simulink model "gm_hybrid_lht_vnl"  (R2019b)
settings: Solver=FixedStepDiscrete  StartTime=0.0  StopTime=inf  FixedStep=1/120e6  RelTol=1e-3
undefined symbols (not defined in the file or in its folder): bt, height, nTheta, width
libraries: hdlsllib x632, simulink x518, hdlmdlgenlib x7, dspsrcs4 x1
(part 2 of 18)

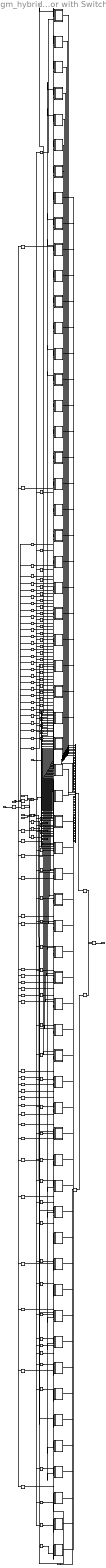
== system gm_hybrid_lht_vnl/Hybrid LHT/Hybrid LHT Accumulator/Accumulator with Switches ==
  shift : Inport  OutDataTypeStr=fixdt(0, 6, 0)  PortDimensions=[1 60]  SampleTime=8.33333333333333e-09
  hough_address : Inport  Port=2  OutDataTypeStr=fixdt(0, 11, 0)  PortDimensions=[1 60]  SampleTime=8.33333333333333e-09
  edge : Inport  Port=3  OutDataTypeStr=boolean  PortDimensions=1  SampleTime=8.33333333333333e-09
  mode : Inport  Port=4  OutDataTypeStr=boolean  PortDimensions=1  SampleTime=8.33333333333333e-09
  read_address : Inport  Port=5  OutDataTypeStr=uint16  PortDimensions=1  SampleTime=8.33333333333333e-09
  clear : Inport  Port=6  OutDataTypeStr=boolean  PortDimensions=1  SampleTime=8.33333333333333e-09
  theta_index : Inport  Port=7  OutDataTypeStr=uint16  PortDimensions=1  SampleTime=8.33333333333333e-09
  Accumulator_instance1 : Subsystem
  Accumulator_instance10 : Subsystem
  Accumulator_instance11 : Subsystem
  Accumulator_instance12 : Subsystem
  Accumulator_instance13 : Subsystem
  Accumulator_instance14 : Subsystem
  Accumulator_instance15 : Subsystem
  Accumulator_instance16 : Subsystem
  Accumulator_instance17 : Subsystem
  Accumulator_instance18 : Subsystem
  Accumulator_instance19 : Subsystem
  Accumulator_instance2 : Subsystem
  Accumulator_instance20 : Subsystem
  Accumulator_instance21 : Subsystem
  Accumulator_instance22 : Subsystem
  Accumulator_instance23 : Subsystem
  Accumulator_instance24 : Subsystem
  Accumulator_instance25 : Subsystem
  Accumulator_instance26 : Subsystem
  Accumulator_instance27 : Subsystem
  Accumulator_instance28 : Subsystem
  Accumulator_instance29 : Subsystem
  Accumulator_instance3 : Subsystem
  Accumulator_instance30 : Subsystem
  Accumulator_instance31 : Subsystem
  Accumulator_instance32 : Subsystem
  Accumulator_instance33 : Subsystem
  Accumulator_instance34 : Subsystem
  Accumulator_instance35 : Subsystem
  Accumulator_instance36 : Subsystem
  Accumulator_instance37 : Subsystem
  Accumulator_instance38 : Subsystem
  Accumulator_instance39 : Subsystem
  Accumulator_instance4 : Subsystem
  Accumulator_instance40 : Subsystem
  Accumulator_instance41 : Subsystem
  Accumulator_instance42 : Subsystem
  Accumulator_instance43 : Subsystem
  Accumulator_instance44 : Subsystem
  Accumulator_instance45 : Subsystem
  Accumulator_instance46 : Subsystem
  Accumulator_instance47 : Subsystem
  Accumulator_instance48 : Subsystem
  Accumulator_instance49 : Subsystem
  Accumulator_instance5 : Subsystem
  Accumulator_instance50 : Subsystem
  Accumulator_instance51 : Subsystem
  Accumulator_instance52 : Subsystem
  Accumulator_instance53 : Subsystem
  Accumulator_instance54 : Subsystem
  Accumulator_instance55 : Subsystem
  Accumulator_instance56 : Subsystem
  Accumulator_instance57 : Subsystem
  Accumulator_instance58 : Subsystem
  Accumulator_instance59 : Subsystem
  Accumulator_instance6 : Subsystem
  Accumulator_instance60 : Subsystem
  Accumulator_instance7 : Subsystem
  Accumulator_instance8 : Subsystem
  Accumulator_instance9 : Subsystem
  Data Type Conversion : DataTypeConversion  OutDataTypeStr=fixdt(0, 11, 0)  SampleTime=8.33333333333333e-09
  Delay : Delay  DelayLength=double(1)  InitialCondition=0  SampleTime=8.33333333333333e-09
  Multiport Switch1 : MultiPortSwitch  DataPortOrder=Zero-based contiguous  Inputs=2  DiagnosticForDefault=None  zeroidx=on  SampleTime=8.33333333333333e-09
  Selector : Selector  NumberOfDimensions=2  IndexMode=Zero-based  SampleTime=8.33333333333333e-09  IndexOptions=Index vector (dialog),Index vector (port)  Indices=double(0),double(0)  OutputSizes=double(1),double(1)
  Switch : Switch  Criteria=u2 > Threshold  Threshold=double(0)  OutDataTypeStr=fixdt(0, 11, 0)  SampleTime=8.33333333333333e-09
  delayMatch{,1..122} (123 alike) : Delay  DelayLength=double(2)  InitialCondition=0  SampleTime=8.33333333333333e-09
  t : Demux  Outputs=60
  t1 : Demux  Outputs=60
  t2 : Concatenate  NumInputs=60
  t3 : Reshape  OutputDimensionality=Row vector (2-D)
  hps : Outport
  wires:
  Delay/1 -> delayMatch122/1
  Multiport Switch1/1 -> delayMatch3/1, delayMatch5/1, delayMatch7/1, delayMatch9/1, delayMatch11/1, delayMatch13/1, delayMatch15/1, delayMatch17/1, delayMatch19/1, delayMatch21/1, delayMatch23/1, delayMatch25/1, delayMatch27/1, delayMatch29/1, delayMatch31/1, delayMatch33/1, delayMatch35/1, delayMatch37/1, delayMatch39/1, delayMatch41/1, delayMatch43/1, delayMatch45/1, delayMatch47/1, delayMatch49/1, delayMatch51/1, delayMatch53/1, delayMatch55/1, delayMatch57/1, delayMatch59/1, delayMatch61/1, delayMatch63/1, delayMatch65/1, delayMatch67/1, delayMatch69/1, delayMatch71/1, delayMatch73/1, delayMatch75/1, delayMatch77/1, delayMatch79/1, delayMatch81/1, delayMatch83/1, delayMatch85/1, delayMatch87/1, delayMatch89/1, delayMatch91/1, delayMatch93/1, delayMatch95/1, delayMatch97/1, delayMatch99/1, delayMatch101/1, delayMatch103/1, delayMatch105/1, delayMatch107/1, delayMatch109/1, delayMatch111/1, delayMatch113/1, delayMatch115/1, delayMatch117/1, delayMatch119/1, delayMatch121/1
  delayMatch121/1 -> Accumulator_instance60/4(edge)
  delayMatch120/1 -> Accumulator_instance60/2(mode)
  delayMatch119/1 -> Accumulator_instance59/4(edge)
  delayMatch118/1 -> Accumulator_instance59/2(mode)
  delayMatch117/1 -> Accumulator_instance58/4(edge)
  delayMatch116/1 -> Accumulator_instance58/2(mode)
  delayMatch115/1 -> Accumulator_instance57/4(edge)
  delayMatch114/1 -> Accumulator_instance57/2(mode)
  delayMatch113/1 -> Accumulator_instance56/4(edge)
  delayMatch112/1 -> Accumulator_instance56/2(mode)
  delayMatch111/1 -> Accumulator_instance55/4(edge)
  delayMatch110/1 -> Accumulator_instance55/2(mode)
  delayMatch109/1 -> Accumulator_instance54/4(edge)
  delayMatch108/1 -> Accumulator_instance54/2(mode)
  delayMatch107/1 -> Accumulator_instance53/4(edge)
  delayMatch106/1 -> Accumulator_instance53/2(mode)
  delayMatch105/1 -> Accumulator_instance52/4(edge)
  delayMatch104/1 -> Accumulator_instance52/2(mode)
  delayMatch103/1 -> Accumulator_instance51/4(edge)
  delayMatch102/1 -> Accumulator_instance51/2(mode)
  delayMatch101/1 -> Accumulator_instance50/4(edge)
  delayMatch100/1 -> Accumulator_instance50/2(mode)
  delayMatch99/1 -> Accumulator_instance49/4(edge)
  delayMatch98/1 -> Accumulator_instance49/2(mode)
  delayMatch97/1 -> Accumulator_instance48/4(edge)
  delayMatch96/1 -> Accumulator_instance48/2(mode)
  delayMatch95/1 -> Accumulator_instance47/4(edge)
  delayMatch94/1 -> Accumulator_instance47/2(mode)
  delayMatch93/1 -> Accumulator_instance46/4(edge)
  delayMatch92/1 -> Accumulator_instance46/2(mode)
  delayMatch91/1 -> Accumulator_instance45/4(edge)
  delayMatch90/1 -> Accumulator_instance45/2(mode)
  delayMatch89/1 -> Accumulator_instance44/4(edge)
  delayMatch88/1 -> Accumulator_instance44/2(mode)
  delayMatch87/1 -> Accumulator_instance43/4(edge)
  delayMatch86/1 -> Accumulator_instance43/2(mode)
  delayMatch85/1 -> Accumulator_instance42/4(edge)
  delayMatch84/1 -> Accumulator_instance42/2(mode)
  delayMatch83/1 -> Accumulator_instance41/4(edge)
  delayMatch82/1 -> Accumulator_instance41/2(mode)
  delayMatch81/1 -> Accumulator_instance40/4(edge)
  delayMatch80/1 -> Accumulator_instance40/2(mode)
  delayMatch79/1 -> Accumulator_instance39/4(edge)
  delayMatch78/1 -> Accumulator_instance39/2(mode)
  delayMatch77/1 -> Accumulator_instance38/4(edge)
  delayMatch76/1 -> Accumulator_instance38/2(mode)
  delayMatch75/1 -> Accumulator_instance37/4(edge)
  delayMatch74/1 -> Accumulator_instance37/2(mode)
  delayMatch73/1 -> Accumulator_instance36/4(edge)
  delayMatch72/1 -> Accumulator_instance36/2(mode)
  delayMatch71/1 -> Accumulator_instance35/4(edge)
  delayMatch70/1 -> Accumulator_instance35/2(mode)
  delayMatch69/1 -> Accumulator_instance34/4(edge)
  delayMatch68/1 -> Accumulator_instance34/2(mode)
  delayMatch67/1 -> Accumulator_instance33/4(edge)
  delayMatch66/1 -> Accumulator_instance33/2(mode)
  delayMatch65/1 -> Accumulator_instance32/4(edge)
  delayMatch64/1 -> Accumulator_instance32/2(mode)
  delayMatch63/1 -> Accumulator_instance31/4(edge)
  delayMatch62/1 -> Accumulator_instance31/2(mode)
  delayMatch61/1 -> Accumulator_instance30/4(edge)
  delayMatch60/1 -> Accumulator_instance30/2(mode)
  delayMatch59/1 -> Accumulator_instance29/4(edge)
  delayMatch58/1 -> Accumulator_instance29/2(mode)
  delayMatch57/1 -> Accumulator_instance28/4(edge)
  delayMatch56/1 -> Accumulator_instance28/2(mode)
  delayMatch55/1 -> Accumulator_instance27/4(edge)
  delayMatch54/1 -> Accumulator_instance27/2(mode)
  delayMatch53/1 -> Accumulator_instance26/4(edge)
  delayMatch52/1 -> Accumulator_instance26/2(mode)
  delayMatch51/1 -> Accumulator_instance25/4(edge)
  delayMatch50/1 -> Accumulator_instance25/2(mode)
  delayMatch49/1 -> Accumulator_instance24/4(edge)
  delayMatch48/1 -> Accumulator_instance24/2(mode)
  delayMatch47/1 -> Accumulator_instance23/4(edge)
  delayMatch46/1 -> Accumulator_instance23/2(mode)
  delayMatch45/1 -> Accumulator_instance22/4(edge)
  delayMatch44/1 -> Accumulator_instance22/2(mode)
  delayMatch43/1 -> Accumulator_instance21/4(edge)
  delayMatch42/1 -> Accumulator_instance21/2(mode)
  delayMatch41/1 -> Accumulator_instance20/4(edge)
  delayMatch40/1 -> Accumulator_instance20/2(mode)
  delayMatch39/1 -> Accumulator_instance19/4(edge)
  delayMatch38/1 -> Accumulator_instance19/2(mode)
  delayMatch37/1 -> Accumulator_instance18/4(edge)
  delayMatch36/1 -> Accumulator_instance18/2(mode)
  delayMatch35/1 -> Accumulator_instance17/4(edge)
  delayMatch34/1 -> Accumulator_instance17/2(mode)
  delayMatch33/1 -> Accumulator_instance16/4(edge)
  delayMatch32/1 -> Accumulator_instance16/2(mode)
  delayMatch31/1 -> Accumulator_instance15/4(edge)
  delayMatch30/1 -> Accumulator_instance15/2(mode)
  delayMatch29/1 -> Accumulator_instance14/4(edge)
  delayMatch28/1 -> Accumulator_instance14/2(mode)
  delayMatch27/1 -> Accumulator_instance13/4(edge)
  delayMatch26/1 -> Accumulator_instance13/2(mode)
  delayMatch25/1 -> Accumulator_instance12/4(edge)
  delayMatch24/1 -> Accumulator_instance12/2(mode)
  delayMatch23/1 -> Accumulator_instance11/4(edge)
  delayMatch22/1 -> Accumulator_instance11/2(mode)
  delayMatch21/1 -> Accumulator_instance10/4(edge)
  delayMatch20/1 -> Accumulator_instance10/2(mode)
  delayMatch19/1 -> Accumulator_instance9/4(edge)
  delayMatch18/1 -> Accumulator_instance9/2(mode)
  delayMatch17/1 -> Accumulator_instance8/4(edge)
  delayMatch16/1 -> Accumulator_instance8/2(mode)
  delayMatch15/1 -> Accumulator_instance7/4(edge)
  delayMatch14/1 -> Accumulator_instance7/2(mode)
  delayMatch13/1 -> Accumulator_instance6/4(edge)
  delayMatch12/1 -> Accumulator_instance6/2(mode)
  delayMatch11/1 -> Accumulator_instance5/4(edge)
  delayMatch10/1 -> Accumulator_instance5/2(mode)
  delayMatch9/1 -> Accumulator_instance4/4(edge)
  delayMatch8/1 -> Accumulator_instance4/2(mode)
  delayMatch7/1 -> Accumulator_instance3/4(edge)
  delayMatch6/1 -> Accumulator_instance3/2(mode)
  delayMatch5/1 -> Accumulator_instance2/4(edge)
  delayMatch4/1 -> Accumulator_instance2/2(mode)
  Data Type Conversion/1 -> delayMatch1/1
  delayMatch2/1 -> Accumulator_instance1/2(mode)
  theta_index/1 -> Delay/1
  clear/1 -> Multiport Switch1/2
  read_address/1 -> Data Type Conversion/1
  mode/1 -> Multiport Switch1/1, delayMatch/1, delayMatch2/1, delayMatch4/1, delayMatch6/1, delayMatch8/1, delayMatch10/1, delayMatch12/1, delayMatch14/1, delayMatch16/1, delayMatch18/1, delayMatch20/1, delayMatch22/1, delayMatch24/1, delayMatch26/1, delayMatch28/1, delayMatch30/1, delayMatch32/1, delayMatch34/1, delayMatch36/1, delayMatch38/1, delayMatch40/1, delayMatch42/1, delayMatch44/1, delayMatch46/1, delayMatch48/1, delayMatch50/1, delayMatch52/1, delayMatch54/1, delayMatch56/1, delayMatch58/1, delayMatch60/1, delayMatch62/1, delayMatch64/1, delayMatch66/1, delayMatch68/1, delayMatch70/1, delayMatch72/1, delayMatch74/1, delayMatch76/1, delayMatch78/1, delayMatch80/1, delayMatch82/1, delayMatch84/1, delayMatch86/1, delayMatch88/1, delayMatch90/1, delayMatch92/1, delayMatch94/1, delayMatch96/1, delayMatch98/1, delayMatch100/1, delayMatch102/1, delayMatch104/1, delayMatch106/1, delayMatch108/1, delayMatch110/1, delayMatch112/1, delayMatch114/1, delayMatch116/1, delayMatch118/1, delayMatch120/1
  edge/1 -> Multiport Switch1/3
  hough_address/1 -> Switch/1
  shift/1 -> t/1
  Accumulator_instance60/1(hps) -> t2/60
  Accumulator_instance59/1(hps) -> t2/59
  Accumulator_instance58/1(hps) -> t2/58
  Accumulator_instance57/1(hps) -> t2/57
  Accumulator_instance56/1(hps) -> t2/56
  Accumulator_instance55/1(hps) -> t2/55
  Accumulator_instance54/1(hps) -> t2/54
  Accumulator_instance53/1(hps) -> t2/53
  Accumulator_instance52/1(hps) -> t2/52
  Accumulator_instance51/1(hps) -> t2/51
  Accumulator_instance50/1(hps) -> t2/50
  Accumulator_instance49/1(hps) -> t2/49
  Accumulator_instance48/1(hps) -> t2/48
  Accumulator_instance47/1(hps) -> t2/47
  Accumulator_instance46/1(hps) -> t2/46
  Accumulator_instance45/1(hps) -> t2/45
  Accumulator_instance44/1(hps) -> t2/44
  Accumulator_instance43/1(hps) -> t2/43
  Accumulator_instance42/1(hps) -> t2/42
  Accumulator_instance41/1(hps) -> t2/41
  Accumulator_instance40/1(hps) -> t2/40
  Accumulator_instance39/1(hps) -> t2/39
  Accumulator_instance38/1(hps) -> t2/38
  Accumulator_instance37/1(hps) -> t2/37
  Accumulator_instance36/1(hps) -> t2/36
  Accumulator_instance35/1(hps) -> t2/35
  Accumulator_instance34/1(hps) -> t2/34
  Accumulator_instance33/1(hps) -> t2/33
  Accumulator_instance32/1(hps) -> t2/32
  Accumulator_instance31/1(hps) -> t2/31
  Accumulator_instance30/1(hps) -> t2/30
  Accumulator_instance29/1(hps) -> t2/29
  Accumulator_instance28/1(hps) -> t2/28
  Accumulator_instance27/1(hps) -> t2/27
  Accumulator_instance26/1(hps) -> t2/26
  Accumulator_instance25/1(hps) -> t2/25
  Accumulator_instance24/1(hps) -> t2/24
  Accumulator_instance23/1(hps) -> t2/23
  Accumulator_instance22/1(hps) -> t2/22
  Accumulator_instance21/1(hps) -> t2/21
  Accumulator_instance20/1(hps) -> t2/20
  Accumulator_instance19/1(hps) -> t2/19
  Accumulator_instance18/1(hps) -> t2/18
  Accumulator_instance17/1(hps) -> t2/17
  Accumulator_instance16/1(hps) -> t2/16
  Accumulator_instance15/1(hps) -> t2/15
  Accumulator_instance14/1(hps) -> t2/14
  Accumulator_instance13/1(hps) -> t2/13
  Accumulator_instance12/1(hps) -> t2/12
  Accumulator_instance11/1(hps) -> t2/11
  Accumulator_instance10/1(hps) -> t2/10
  Accumulator_instance9/1(hps) -> t2/9
  Accumulator_instance8/1(hps) -> t2/8
  Accumulator_instance7/1(hps) -> t2/7
  Accumulator_instance6/1(hps) -> t2/6
  Accumulator_instance5/1(hps) -> t2/5
  Accumulator_instance4/1(hps) -> t2/4
  Accumulator_instance3/1(hps) -> t2/3
  Accumulator_instance2/1(hps) -> t2/2
  Accumulator_instance1/1(hps) -> t2/1
  t2/1 -> t3/1
  t1/60 -> Accumulator_instance60/3(address)
  t1/59 -> Accumulator_instance59/3(address)
  t1/58 -> Accumulator_instance58/3(address)
  t1/57 -> Accumulator_instance57/3(address)
  t1/56 -> Accumulator_instance56/3(address)
  t1/55 -> Accumulator_instance55/3(address)
  t1/54 -> Accumulator_instance54/3(address)
  t1/53 -> Accumulator_instance53/3(address)
  t1/52 -> Accumulator_instance52/3(address)
  t1/51 -> Accumulator_instance51/3(address)
  t1/50 -> Accumulator_instance50/3(address)
  t1/49 -> Accumulator_instance49/3(address)
  t1/48 -> Accumulator_instance48/3(address)
  t1/47 -> Accumulator_instance47/3(address)
  t1/46 -> Accumulator_instance46/3(address)
  t1/45 -> Accumulator_instance45/3(address)
  t1/44 -> Accumulator_instance44/3(address)
  t1/43 -> Accumulator_instance43/3(address)
  t1/42 -> Accumulator_instance42/3(address)
  t1/41 -> Accumulator_instance41/3(address)
  t1/40 -> Accumulator_instance40/3(address)
  t1/39 -> Accumulator_instance39/3(address)
  t1/38 -> Accumulator_instance38/3(address)
  t1/37 -> Accumulator_instance37/3(address)
  t1/36 -> Accumulator_instance36/3(address)
  t1/35 -> Accumulator_instance35/3(address)
  t1/34 -> Accumulator_instance34/3(address)
  t1/33 -> Accumulator_instance33/3(address)
  t1/32 -> Accumulator_instance32/3(address)
  t1/31 -> Accumulator_instance31/3(address)
  t1/30 -> Accumulator_instance30/3(address)
  t1/29 -> Accumulator_instance29/3(address)
  t1/28 -> Accumulator_instance28/3(address)
  t1/27 -> Accumulator_instance27/3(address)
  t1/26 -> Accumulator_instance26/3(address)
  t1/25 -> Accumulator_instance25/3(address)
  t1/24 -> Accumulator_instance24/3(address)
  t1/23 -> Accumulator_instance23/3(address)
  t1/22 -> Accumulator_instance22/3(address)
  t1/21 -> Accumulator_instance21/3(address)
  t1/20 -> Accumulator_instance20/3(address)
  t1/19 -> Accumulator_instance19/3(address)
  t1/18 -> Accumulator_instance18/3(address)
  t1/17 -> Accumulator_instance17/3(address)
  t1/16 -> Accumulator_instance16/3(address)
  t1/15 -> Accumulator_instance15/3(address)
  t1/14 -> Accumulator_instance14/3(address)
  t1/13 -> Accumulator_instance13/3(address)
  t1/12 -> Accumulator_instance12/3(address)
  t1/11 -> Accumulator_instance11/3(address)
  t1/10 -> Accumulator_instance10/3(address)
  t1/9 -> Accumulator_instance9/3(address)
  t1/8 -> Accumulator_instance8/3(address)
  t1/7 -> Accumulator_instance7/3(address)
  t1/6 -> Accumulator_instance6/3(address)
  t1/5 -> Accumulator_instance5/3(address)
  t1/4 -> Accumulator_instance4/3(address)
  t1/3 -> Accumulator_instance3/3(address)
  t1/2 -> Accumulator_instance2/3(address)
  t1/1 -> Accumulator_instance1/3(address)
  t/60 -> Accumulator_instance60/1(shift)
  t/59 -> Accumulator_instance59/1(shift)
  t/58 -> Accumulator_instance58/1(shift)
  t/57 -> Accumulator_instance57/1(shift)
  t/56 -> Accumulator_instance56/1(shift)
  t/55 -> Accumulator_instance55/1(shift)
  t/54 -> Accumulator_instance54/1(shift)
  t/53 -> Accumulator_instance53/1(shift)
  t/52 -> Accumulator_instance52/1(shift)
  t/51 -> Accumulator_instance51/1(shift)
  t/50 -> Accumulator_instance50/1(shift)
  t/49 -> Accumulator_instance49/1(shift)
  t/48 -> Accumulator_instance48/1(shift)
  t/47 -> Accumulator_instance47/1(shift)
  t/46 -> Accumulator_instance46/1(shift)
  t/45 -> Accumulator_instance45/1(shift)
  t/44 -> Accumulator_instance44/1(shift)
  t/43 -> Accumulator_instance43/1(shift)
  t/42 -> Accumulator_instance42/1(shift)
  t/41 -> Accumulator_instance41/1(shift)
  t/40 -> Accumulator_instance40/1(shift)
  t/39 -> Accumulator_instance39/1(shift)
  t/38 -> Accumulator_instance38/1(shift)
  t/37 -> Accumulator_instance37/1(shift)
  t/36 -> Accumulator_instance36/1(shift)
  t/35 -> Accumulator_instance35/1(shift)
  t/34 -> Accumulator_instance34/1(shift)
  t/33 -> Accumulator_instance33/1(shift)
  t/32 -> Accumulator_instance32/1(shift)
  t/31 -> Accumulator_instance31/1(shift)
  t/30 -> Accumulator_instance30/1(shift)
  t/29 -> Accumulator_instance29/1(shift)
  t/28 -> Accumulator_instance28/1(shift)
  t/27 -> Accumulator_instance27/1(shift)
  t/26 -> Accumulator_instance26/1(shift)
  t/25 -> Accumulator_instance25/1(shift)
  t/24 -> Accumulator_instance24/1(shift)
  t/23 -> Accumulator_instance23/1(shift)
  t/22 -> Accumulator_instance22/1(shift)
  t/21 -> Accumulator_instance21/1(shift)
  t/20 -> Accumulator_instance20/1(shift)
  t/19 -> Accumulator_instance19/1(shift)
  t/18 -> Accumulator_instance18/1(shift)
  t/17 -> Accumulator_instance17/1(shift)
  t/16 -> Accumulator_instance16/1(shift)
  t/15 -> Accumulator_instance15/1(shift)
  t/14 -> Accumulator_instance14/1(shift)
  t/13 -> Accumulator_instance13/1(shift)
  t/12 -> Accumulator_instance12/1(shift)
  t/11 -> Accumulator_instance11/1(shift)
  t/10 -> Accumulator_instance10/1(shift)
  t/9 -> Accumulator_instance9/1(shift)
  t/8 -> Accumulator_instance8/1(shift)
  t/7 -> Accumulator_instance7/1(shift)
  t/6 -> Accumulator_instance6/1(shift)
  t/5 -> Accumulator_instance5/1(shift)
  t/4 -> Accumulator_instance4/1(shift)
  t/3 -> Accumulator_instance3/1(shift)
  t/2 -> Accumulator_instance2/1(shift)
  t/1 -> Accumulator_instance1/1(shift)
  Switch/1 -> t1/1
  Selector/1 -> hps/1
  delayMatch3/1 -> Accumulator_instance1/4(edge)
  delayMatch122/1 -> Selector/2
  delayMatch1/1 -> Switch/3
  t3/1 -> Selector/1
  delayMatch/1 -> Switch/2

== system gm_hybrid_lht_vnl/Hybrid LHT/Hybrid LHT Kernel/Extract Active Votes ==
  note: Check the indices to ensure they are in the correct limits
  Theta : Inport  OutDataTypeStr=uint8  PortDimensions=1  SampleTime=8.33333333333333e-09
  Add : Sum  AccumDataTypeStr=fixdt(1, 10, 0)  OutDataTypeStr=fixdt(1, 10, 0)  SampleTime=8.33333333333333e-09
  Add1 : Sum  Inputs=+-  AccumDataTypeStr=fixdt(1, 12, 0)  OutDataTypeStr=fixdt(1, 12, 0)  SampleTime=8.33333333333333e-09
  Add2 : Sum  Inputs=+-  AccumDataTypeStr=fixdt(1, 9, 0)  OutDataTypeStr=fixdt(1, 9, 0)  SampleTime=8.33333333333333e-09
  Add3 : Sum  AccumDataTypeStr=fixdt(1, 11, 0)  OutDataTypeStr=fixdt(1, 11, 0)  SampleTime=8.33333333333333e-09
  Add4 : Sum  Inputs=+-  AccumDataTypeStr=uint8  OutDataTypeStr=uint8  SampleTime=8.33333333333333e-09
  Constant : Constant  Value=[-30 -29 -28 -27 -26 -25 -24 -23 -22 -21 -20 -19 -18 -17 -16 -15 -14 -13 -12 -11 -10 -9 -8 -7 -6 -5 -4 -3 -2 -1 0 1 2 3 4 5 6 7 8 9 10 11 12 13 14 15 16 17 18 19 20 21 22 23 24 25 26 27 28 29]  VectorParams1D=off  OutDataTypeStr=fixdt(1, 6, 0)  SampleTime=-1
  Data Type Conversion : DataTypeConversion  OutDataTypeStr=uint8  SampleTime=8.33333333333333e-09
  Data Type Conversion1 : DataTypeConversion  OutDataTypeStr=uint8  SampleTime=8.33333333333333e-09
  Gain1 : Product  Inputs=**  OutDataTypeStr=uint8  SampleTime=8.33333333333333e-09
  Gain1_const : Constant  Value=60  OutDataTypeStr=uint8  SampleTime=-1
  GetShift : Subsystem
  High : Constant  Value=59  OutDataTypeStr=uint8  SampleTime=-1
  High1 : Constant  Value=59  OutDataTypeStr=uint8  SampleTime=-1
  Low : Constant  Value=0  OutDataTypeStr=fixdt(0, 1, 0)  SampleTime=-1
  Multiport Switch2 : MultiPortSwitch  DataPortOrder=Zero-based contiguous  Inputs=2  DiagnosticForDefault=None  zeroidx=on  OutDataTypeStr=fixdt(1, 11, 0)  SampleTime=8.33333333333333e-09
  Multiport Switch3 : MultiPortSwitch  DataPortOrder=Zero-based contiguous  Inputs=2  DiagnosticForDefault=None  zeroidx=on  OutDataTypeStr=fixdt(1, 12, 0)  SampleTime=8.33333333333333e-09
  PipelineRegister : Delay  DelayLength=double(1)  InitialCondition=0  SampleTime=8.33333333333333e-09
  Relational : RelationalOperator  Operator=<  OutDataTypeStr=boolean  SampleTime=8.33333333333333e-09  RndMeth=Nearest
  Relational1 : RelationalOperator  Operator=>  OutDataTypeStr=boolean  SampleTime=8.33333333333333e-09  RndMeth=Nearest
  Selector4 : Selector  NumberOfDimensions=2  IndexMode=Zero-based  SampleTime=8.33333333333333e-09  IndexOptions=Index vector (dialog),Index vector (dialog)  Indices=double(0),double([59 58 57 56 55 54 53 52 51 50 49 48 47 46 45 44 43 42 41 40 39 38 37 36 35 34 33 32 31 30 29 28 27 26 25 24 23 22 21 20 19 18 17 16 15 14 13 12 11 10 9 8 7 6 5 4 3 2 1 0])  OutputSizes=double(1),double(1)
  delayMatch : Delay  DelayLength=double(1)  InitialCondition=0  SampleTime=8.33333333333333e-09
  nTheta : Constant  Value=60  OutDataTypeStr=uint8  SampleTime=-1
  Index : Outport  VectorParamsAs1DForOutWhenUnconnected=off
  wires:
  Gain1/1 -> PipelineRegister/1
  Theta/1 -> GetShift/1(Theta), delayMatch/1
  Gain1_const/1 -> Gain1/1
  nTheta/1 -> Add1/2, Add3/2
  Selector4/1 -> Index/1
  Relational1/1 -> Multiport Switch3/1
  Relational/1 -> Multiport Switch2/1
  Multiport Switch3/1 -> Data Type Conversion/1
  Multiport Switch2/1 -> Add1/1, Multiport Switch3/2, Relational1/1
  Low/1 -> Relational/2
  High1/1 -> Add4/1
  High/1 -> Relational1/2
  GetShift/1(Shift) -> Gain1/2
  PipelineRegister/1 -> Add2/2
  Data Type Conversion1/1 -> Add4/2
  Data Type Conversion/1 -> Data Type Conversion1/1
  Constant/1 -> Add/2
  Add4/1 -> Selector4/1
  Add3/1 -> Multiport Switch2/3
  Add2/1 -> Add/1
  Add1/1 -> Multiport Switch3/3
  Add/1 -> Add3/1, Multiport Switch2/2, Relational/1
  delayMatch/1 -> Add2/1

== system gm_hybrid_lht_vnl/Hybrid LHT/Hybrid LHT Kernel/Gradient Kernel System ==
  Edge : Inport  OutDataTypeStr=fixdt(0, 1, 0)  PortDimensions=1  SampleTime=8.33333333333333e-09
  X : Inport  Port=2  OutDataTypeStr=fixdt(1, 11, 0)  PortDimensions=1  SampleTime=8.33333333333333e-09
  Y : Inport  Port=3  OutDataTypeStr=fixdt(1, 10, 0)  PortDimensions=1  SampleTime=8.33333333333333e-09
  Theta : Inport  Port=4  OutDataTypeStr=uint8  PortDimensions=1  SampleTime=8.33333333333333e-09
  Get Index and Fix Limits : Subsystem
  Hough Kernel : Subsystem
  vEdge : Outport  VectorParamsAs1DForOutWhenUnconnected=off
  Rho : Outport  Port=2  VectorParamsAs1DForOutWhenUnconnected=off
  Shift : Outport  Port=3  VectorParamsAs1DForOutWhenUnconnected=off
  wires:
  Theta/1 -> Get Index and Fix Limits/1(Theta)
  Y/1 -> Hough Kernel/3(Y)
  X/1 -> Hough Kernel/2(X)
  Edge/1 -> Hough Kernel/1(Edge)
  Hough Kernel/2(Rho) -> Rho/1
  Hough Kernel/1(vEdge) -> vEdge/1
  Get Index and Fix Limits/2(Shift) -> Shift/1
  Get Index and Fix Limits/1(Index) -> Hough Kernel/4(Index)

== system gm_hybrid_lht_vnl/Hybrid LHT_vnl/Hybrid LHT Accumulator/Accumulator with Switches ==
  shift : Inport
  hough_address : Inport  Port=2
  edge : Inport  Port=3
  mode : Inport  Port=4
  read_address : Inport  Port=5
  clear : Inport  Port=6
  theta_index : Inport  Port=7
  Accumulator : Subsystem
  Data Type Conversion : DataTypeConversion  OutDataTypeStr=fixdt(0,ceil(log2(maxRho*2)),0)
  Delay : Delay  DelayLength=1
  Multiport Switch1 : MultiPortSwitch  DataPortOrder=Zero-based contiguous  Inputs=2  zeroidx=on
  Selector : Selector  NumberOfDimensions=2  IndexMode=Zero-based  InputPortWidth=3  IndexOptions=Index vector (dialog),Index vector (port)  Indices=0,0  OutputSizes=1,1
  Switch : Switch  Criteria=u2 > Threshold
  hps : Outport
  wires:
  shift/1 -> Accumulator/1(shift)
  Accumulator/1(hps) -> Selector/1
  mode/1 -> Switch/2, Multiport Switch1/1, Accumulator/2(mode)
  read_address/1 -> Data Type Conversion/1
  Switch/1 -> Accumulator/3(address)
  Multiport Switch1/1 -> Accumulator/4(edge)
  hough_address/1 -> Switch/1
  theta_index/1 -> Delay/1
  Selector/1 -> hps/1
  edge/1 -> Multiport Switch1/3
  clear/1 -> Multiport Switch1/2
  Data Type Conversion/1 -> Switch/3
  Delay/1 -> Selector/2

== system gm_hybrid_lht_vnl/Hybrid LHT_vnl/Hybrid LHT Kernel/Extract Active Votes ==
  note: Check the indices to ensure they are in the correct limits
  Theta : Inport
  Add : Sum
  Add1 : Sum  Inputs=+-
  Add2 : Sum  Inputs=+-
  Add3 : Sum
  Add4 : Sum  Inputs=+-  OutDataTypeStr=uint8
  Constant : Constant  Value=[-lambda:1:lambda-subflag]  VectorParams1D=off  OutDataTypeStr=fixdt(1,ceil(log2(lambda+1))+1, 0)  SampleTime=-1
  Data Type Conversion : DataTypeConversion  OutDataTypeStr=fixdt(0, ceil(log2(nTheta+1)), 0)
  Data Type Conversion1 : DataTypeConversion  OutDataTypeStr=uint8
  Gain1 : Gain  Gain=nTheta/L  ParamDataTypeStr=fixdt(0, ceil(log2(nTheta+1)), 0)  OutDataTypeStr=fixdt(0, ceil(log2(nTheta+1)), 0)
  GetShift : Subsystem
  High : Constant  Value=nTheta/L-1  OutDataTypeStr=fixdt(0,ceil(log2(nTheta)),0)  SampleTime=-1
  High1 : Constant  Value=nTheta/L-1  OutDataTypeStr=fixdt(0,ceil(log2(nTheta)),0)  SampleTime=-1
  Low : Constant  Value=0  OutDataTypeStr=fixdt(0,1,0)  SampleTime=-1
  Multiport Switch2 : MultiPortSwitch  DataPortOrder=Zero-based contiguous  Inputs=2  zeroidx=on
  Multiport Switch3 : MultiPortSwitch  DataPortOrder=Zero-based contiguous  Inputs=2  zeroidx=on
  Relational : RelationalOperator  Operator=<  OutDataTypeStr=boolean  RndMeth=Nearest
  Relational1 : RelationalOperator  Operator=>  OutDataTypeStr=boolean  RndMeth=Nearest
  Selector4 : Selector  NumberOfDimensions=2  IndexMode=Zero-based  InputPortWidth=3  IndexOptions=Index vector (dialog),Index vector (dialog)  Indices=0,[nTheta/floor(36/ceil(log2(2*maxRho)))-1:-1:0]  OutputSizes=1,1
  nTheta : Constant  Value=nTheta/L  OutDataTypeStr=fixdt(0,ceil(log2(nTheta+1)),0)  SampleTime=-1
  Index : Outport  VectorParamsAs1DForOutWhenUnconnected=off
  wires:
  Gain1/1 -> Add2/2
  GetShift/1(Shift) -> Gain1/1
  Selector4/1 -> Index/1
  Constant/1 -> Add/2
  Add1/1 -> Multiport Switch3/3
  Relational/1 -> Multiport Switch2/1
  Multiport Switch3/1 -> Data Type Conversion/1
  High/1 -> Relational1/2
  Relational1/1 -> Multiport Switch3/1
  Add3/1 -> Multiport Switch2/3
  Low/1 -> Relational/2
  Multiport Switch2/1 -> Add1/1, Relational1/1, Multiport Switch3/2
  nTheta/1 -> Add3/2, Add1/2
  Theta/1 -> Add2/1, GetShift/1(Theta)
  Add/1 -> Add3/1, Relational/1, Multiport Switch2/2
  Add2/1 -> Add/1
  High1/1 -> Add4/1
  Add4/1 -> Selector4/1
  Data Type Conversion/1 -> Data Type Conversion1/1
  Data Type Conversion1/1 -> Add4/2

== system gm_hybrid_lht_vnl/Hybrid LHT_vnl/Hybrid LHT Kernel/Gradient Kernel System ==
  Edge : Inport
  X : Inport  Port=2
  Y : Inport  Port=3
  Theta : Inport  Port=4
  Get Index and Fix Limits : Subsystem  TreatAsAtomicUnit=on
  Hough Kernel : Subsystem  VariantControl=Simple
  vEdge : Outport  VectorParamsAs1DForOutWhenUnconnected=off
  Rho : Outport  Port=2  VectorParamsAs1DForOutWhenUnconnected=off
  Shift : Outport  Port=3  VectorParamsAs1DForOutWhenUnconnected=off
  wires:
  Get Index and Fix Limits/2(Shift) -> Shift/1
  Hough Kernel/2(Rho) -> Rho/1
  Hough Kernel/1(vEdge) -> vEdge/1
  Edge/1 -> Hough Kernel/1(Edge)
  X/1 -> Hough Kernel/2(X)
  Y/1 -> Hough Kernel/3(Y)
  Theta/1 -> Get Index and Fix Limits/1(Theta)
  Get Index and Fix Limits/1(Index) -> Hough Kernel/4(Index)

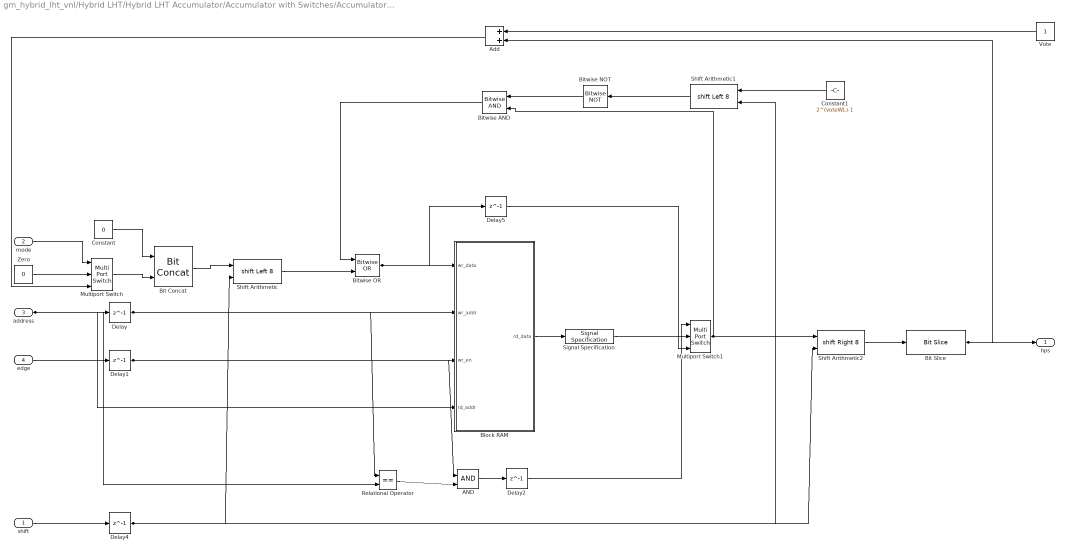
== system gm_hybrid_lht_vnl/Hybrid LHT/Hybrid LHT Accumulator/Accumulator with Switches/Accumulator_instance1 ==
  shift : Inport  OutDataTypeStr=fixdt(0, 6, 0)  PortDimensions=1  SampleTime=8.33333333333333e-09
  mode : Inport  Port=2  OutDataTypeStr=boolean  PortDimensions=1  SampleTime=8.33333333333333e-09
  address : Inport  Port=3  OutDataTypeStr=fixdt(0, 11, 0)  PortDimensions=1  SampleTime=8.33333333333333e-09
  edge : Inport  Port=4  OutDataTypeStr=boolean  PortDimensions=1  SampleTime=8.33333333333333e-09
  AND : Logic  IconShape=distinctive  AllPortsSameDT=off  OutDataTypeStr=boolean
  Add : Sum  OutDataTypeStr=fixdt(0, ceil(log2(maxRho*2)), 0)
  Bit Concat : hdlsllib/Logic and Bit Operations/Bit Concat  numInputs=2
      settings: SourceProductName=Simulink
  Bit Slice : hdlsllib/Logic and Bit Operations/Bit Slice  lidx=voteWL-1  ridx=0
  Bitwise AND : simulink/Logic and Bit Operations/Bitwise Operator  logicop=AND  UseBitMask=off  NumInputPorts=2  BitMask=bin2dec('11011001')  BitMaskRealWorld=Stored Integer
  Bitwise NOT : simulink/Logic and Bit Operations/Bitwise Operator  logicop=NOT  UseBitMask=off  BitMask=bin2dec('11011001')  BitMaskRealWorld=Stored Integer
  Bitwise OR : simulink/Logic and Bit Operations/Bitwise Operator  logicop=OR  UseBitMask=off  NumInputPorts=2  BitMask=bin2dec('11011001')  BitMaskRealWorld=Stored Integer
  Block RAM : Subsystem
  Constant : Constant  Value=0  OutDataTypeStr=fixdt(0, 36-voteWL, 0)  SampleTime=-1
  Constant1 : Constant  Value=2^(voteWL)-1  OutDataTypeStr=fixdt(0, 36, 0)  SampleTime=-1
  Delay{,1..2,4..5} (5 alike) : Delay  DelayLength=1
  Multiport Switch : MultiPortSwitch  DataPortOrder=Zero-based contiguous  Inputs=2  zeroidx=on
  Multiport Switch1 : MultiPortSwitch  DataPortOrder=Zero-based contiguous  Inputs=2  zeroidx=on
  Relational Operator : RelationalOperator  Operator===  OutDataTypeStr=boolean  RndMeth=Simplest
  Shift Arithmetic : ArithShift  BitShiftNumberSource=Input port  BitShiftNumber=8  BitShiftDirection=Left  DiagnosticForOORShift=Error
      settings: InputPortMap=u0,p1
  Shift Arithmetic1 : ArithShift  BitShiftNumberSource=Input port  BitShiftNumber=8  BitShiftDirection=Left  DiagnosticForOORShift=Error
      settings: InputPortMap=u0,p1
  Shift Arithmetic2 : ArithShift  BitShiftNumberSource=Input port  BitShiftNumber=8  BitShiftDirection=Right  DiagnosticForOORShift=Error
      settings: InputPortMap=u0,p1
  Signal Specification : SignalSpecification  OutDataTypeStr=fixdt(0, 36, 0)
  Vote : Constant  OutDataTypeStr=fixdt(0,1,0)  SampleTime=-1
  Zero : Constant  Value=0  OutDataTypeStr=fixdt(0,1,0)  SampleTime=-1
  hps : Outport
  wires:
  Block RAM/1(rd_data) -> Signal Specification/1
  Multiport Switch1/1 -> Shift Arithmetic2/1, Bitwise AND/2
  Signal Specification/1 -> Multiport Switch1/2
  Bitwise OR/1 -> Block RAM/1(wr_data), Delay5/1
  Bitwise AND/1 -> Bitwise OR/1
  Shift Arithmetic2/1 -> Bit Slice/1
  Add/1 -> Multiport Switch/3
  Multiport Switch/1 -> Bit Concat/2
  Bit Concat/1 -> Shift Arithmetic/1
  Shift Arithmetic/1 -> Bitwise OR/2
  Delay5/1 -> Multiport Switch1/3
  edge/1 -> Delay1/1
  address/1 -> Block RAM/4(rd_addr), Delay/1, Relational Operator/2
  mode/1 -> Multiport Switch/1
  shift/1 -> Delay4/1
  AND/1 -> Delay2/1
  Bit Slice/1 -> Add/2, hps/1
  Bitwise NOT/1 -> Bitwise AND/1
  Constant/1 -> Bit Concat/1
  Constant1/1 -> Shift Arithmetic1/1
  Delay/1 -> Block RAM/2(wr_addr), Relational Operator/1
  Delay1/1 -> Block RAM/3(wr_en), AND/1
  Delay2/1 -> Multiport Switch1/1
  Delay4/1 -> Shift Arithmetic2/2, Shift Arithmetic/2, Shift Arithmetic1/2
  Relational Operator/1 -> AND/2
  Shift Arithmetic1/1 -> Bitwise NOT/1
  Vote/1 -> Add/1
  Zero/1 -> Multiport Switch/2

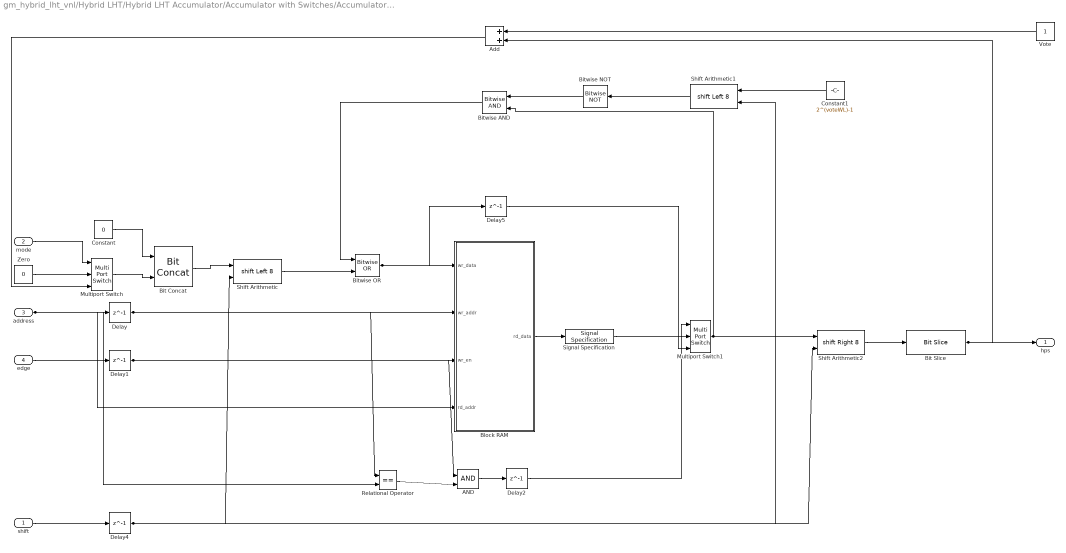
== system gm_hybrid_lht_vnl/Hybrid LHT/Hybrid LHT Accumulator/Accumulator with Switches/Accumulator_instance10 ==
  shift : Inport  OutDataTypeStr=fixdt(0, 6, 0)  PortDimensions=1  SampleTime=8.33333333333333e-09
  mode : Inport  Port=2  OutDataTypeStr=boolean  PortDimensions=1  SampleTime=8.33333333333333e-09
  address : Inport  Port=3  OutDataTypeStr=fixdt(0, 11, 0)  PortDimensions=1  SampleTime=8.33333333333333e-09
  edge : Inport  Port=4  OutDataTypeStr=boolean  PortDimensions=1  SampleTime=8.33333333333333e-09
  AND : Logic  IconShape=distinctive  AllPortsSameDT=off  OutDataTypeStr=boolean
  Add : Sum  OutDataTypeStr=fixdt(0, ceil(log2(maxRho*2)), 0)
  Bit Concat : hdlsllib/Logic and Bit Operations/Bit Concat  numInputs=2
      settings: SourceProductName=Simulink
  Bit Slice : hdlsllib/Logic and Bit Operations/Bit Slice  lidx=voteWL-1  ridx=0
  Bitwise AND : simulink/Logic and Bit Operations/Bitwise Operator  logicop=AND  UseBitMask=off  NumInputPorts=2  BitMask=bin2dec('11011001')  BitMaskRealWorld=Stored Integer
  Bitwise NOT : simulink/Logic and Bit Operations/Bitwise Operator  logicop=NOT  UseBitMask=off  BitMask=bin2dec('11011001')  BitMaskRealWorld=Stored Integer
  Bitwise OR : simulink/Logic and Bit Operations/Bitwise Operator  logicop=OR  UseBitMask=off  NumInputPorts=2  BitMask=bin2dec('11011001')  BitMaskRealWorld=Stored Integer
  Block RAM : Subsystem
  Constant : Constant  Value=0  OutDataTypeStr=fixdt(0, 36-voteWL, 0)  SampleTime=-1
  Constant1 : Constant  Value=2^(voteWL)-1  OutDataTypeStr=fixdt(0, 36, 0)  SampleTime=-1
  Delay{,1..2,4..5} (5 alike) : Delay  DelayLength=1
  Multiport Switch : MultiPortSwitch  DataPortOrder=Zero-based contiguous  Inputs=2  zeroidx=on
  Multiport Switch1 : MultiPortSwitch  DataPortOrder=Zero-based contiguous  Inputs=2  zeroidx=on
  Relational Operator : RelationalOperator  Operator===  OutDataTypeStr=boolean  RndMeth=Simplest
  Shift Arithmetic : ArithShift  BitShiftNumberSource=Input port  BitShiftNumber=8  BitShiftDirection=Left  DiagnosticForOORShift=Error
      settings: InputPortMap=u0,p1
  Shift Arithmetic1 : ArithShift  BitShiftNumberSource=Input port  BitShiftNumber=8  BitShiftDirection=Left  DiagnosticForOORShift=Error
      settings: InputPortMap=u0,p1
  Shift Arithmetic2 : ArithShift  BitShiftNumberSource=Input port  BitShiftNumber=8  BitShiftDirection=Right  DiagnosticForOORShift=Error
      settings: InputPortMap=u0,p1
  Signal Specification : SignalSpecification  OutDataTypeStr=fixdt(0, 36, 0)
  Vote : Constant  OutDataTypeStr=fixdt(0,1,0)  SampleTime=-1
  Zero : Constant  Value=0  OutDataTypeStr=fixdt(0,1,0)  SampleTime=-1
  hps : Outport
  wires:
  Zero/1 -> Multiport Switch/2
  Vote/1 -> Add/1
  Shift Arithmetic1/1 -> Bitwise NOT/1
  Relational Operator/1 -> AND/2
  Delay4/1 -> Shift Arithmetic1/2, Shift Arithmetic/2, Shift Arithmetic2/2
  Delay2/1 -> Multiport Switch1/1
  Delay1/1 -> AND/1, Block RAM/3(wr_en)
  Delay/1 -> Relational Operator/1, Block RAM/2(wr_addr)
  Constant1/1 -> Shift Arithmetic1/1
  Constant/1 -> Bit Concat/1
  Bitwise NOT/1 -> Bitwise AND/1
  Bit Slice/1 -> hps/1, Add/2
  AND/1 -> Delay2/1
  shift/1 -> Delay4/1
  mode/1 -> Multiport Switch/1
  address/1 -> Relational Operator/2, Delay/1, Block RAM/4(rd_addr)
  edge/1 -> Delay1/1
  Delay5/1 -> Multiport Switch1/3
  Shift Arithmetic/1 -> Bitwise OR/2
  Bit Concat/1 -> Shift Arithmetic/1
  Multiport Switch/1 -> Bit Concat/2
  Add/1 -> Multiport Switch/3
  Shift Arithmetic2/1 -> Bit Slice/1
  Bitwise AND/1 -> Bitwise OR/1
  Bitwise OR/1 -> Delay5/1, Block RAM/1(wr_data)
  Signal Specification/1 -> Multiport Switch1/2
  Multiport Switch1/1 -> Bitwise AND/2, Shift Arithmetic2/1
  Block RAM/1(rd_data) -> Signal Specification/1

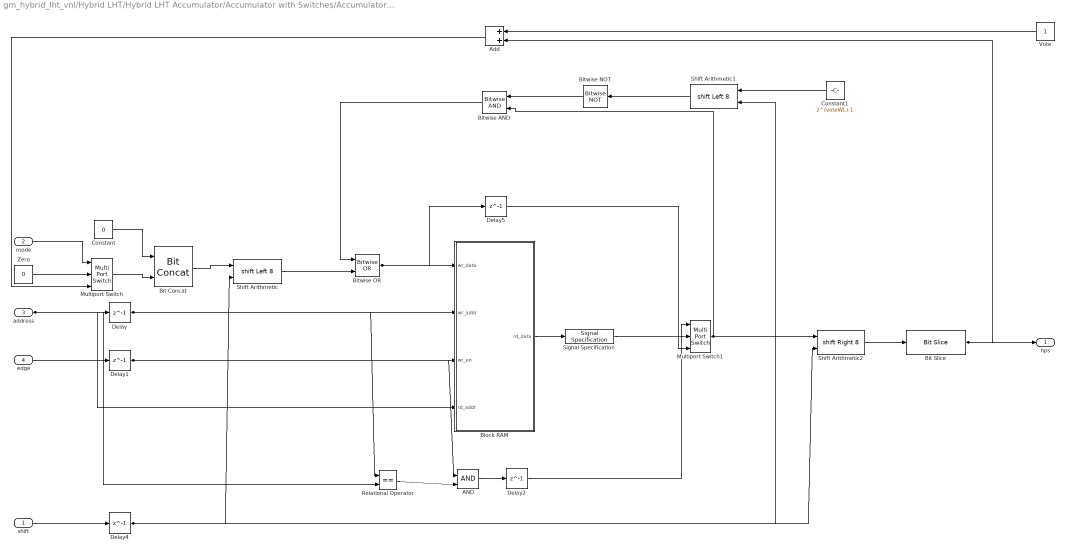
== system gm_hybrid_lht_vnl/Hybrid LHT/Hybrid LHT Accumulator/Accumulator with Switches/Accumulator_instance11 ==
  shift : Inport  OutDataTypeStr=fixdt(0, 6, 0)  PortDimensions=1  SampleTime=8.33333333333333e-09
  mode : Inport  Port=2  OutDataTypeStr=boolean  PortDimensions=1  SampleTime=8.33333333333333e-09
  address : Inport  Port=3  OutDataTypeStr=fixdt(0, 11, 0)  PortDimensions=1  SampleTime=8.33333333333333e-09
  edge : Inport  Port=4  OutDataTypeStr=boolean  PortDimensions=1  SampleTime=8.33333333333333e-09
  AND : Logic  IconShape=distinctive  AllPortsSameDT=off  OutDataTypeStr=boolean
  Add : Sum  OutDataTypeStr=fixdt(0, ceil(log2(maxRho*2)), 0)
  Bit Concat : hdlsllib/Logic and Bit Operations/Bit Concat  numInputs=2
      settings: SourceProductName=Simulink
  Bit Slice : hdlsllib/Logic and Bit Operations/Bit Slice  lidx=voteWL-1  ridx=0
  Bitwise AND : simulink/Logic and Bit Operations/Bitwise Operator  logicop=AND  UseBitMask=off  NumInputPorts=2  BitMask=bin2dec('11011001')  BitMaskRealWorld=Stored Integer
  Bitwise NOT : simulink/Logic and Bit Operations/Bitwise Operator  logicop=NOT  UseBitMask=off  BitMask=bin2dec('11011001')  BitMaskRealWorld=Stored Integer
  Bitwise OR : simulink/Logic and Bit Operations/Bitwise Operator  logicop=OR  UseBitMask=off  NumInputPorts=2  BitMask=bin2dec('11011001')  BitMaskRealWorld=Stored Integer
  Block RAM : Subsystem
  Constant : Constant  Value=0  OutDataTypeStr=fixdt(0, 36-voteWL, 0)  SampleTime=-1
  Constant1 : Constant  Value=2^(voteWL)-1  OutDataTypeStr=fixdt(0, 36, 0)  SampleTime=-1
  Delay{,1..2,4..5} (5 alike) : Delay  DelayLength=1
  Multiport Switch : MultiPortSwitch  DataPortOrder=Zero-based contiguous  Inputs=2  zeroidx=on
  Multiport Switch1 : MultiPortSwitch  DataPortOrder=Zero-based contiguous  Inputs=2  zeroidx=on
  Relational Operator : RelationalOperator  Operator===  OutDataTypeStr=boolean  RndMeth=Simplest
  Shift Arithmetic : ArithShift  BitShiftNumberSource=Input port  BitShiftNumber=8  BitShiftDirection=Left  DiagnosticForOORShift=Error
      settings: InputPortMap=u0,p1
  Shift Arithmetic1 : ArithShift  BitShiftNumberSource=Input port  BitShiftNumber=8  BitShiftDirection=Left  DiagnosticForOORShift=Error
      settings: InputPortMap=u0,p1
  Shift Arithmetic2 : ArithShift  BitShiftNumberSource=Input port  BitShiftNumber=8  BitShiftDirection=Right  DiagnosticForOORShift=Error
      settings: InputPortMap=u0,p1
  Signal Specification : SignalSpecification  OutDataTypeStr=fixdt(0, 36, 0)
  Vote : Constant  OutDataTypeStr=fixdt(0,1,0)  SampleTime=-1
  Zero : Constant  Value=0  OutDataTypeStr=fixdt(0,1,0)  SampleTime=-1
  hps : Outport
  wires:
  Zero/1 -> Multiport Switch/2
  Vote/1 -> Add/1
  Shift Arithmetic1/1 -> Bitwise NOT/1
  Relational Operator/1 -> AND/2
  Delay4/1 -> Shift Arithmetic1/2, Shift Arithmetic/2, Shift Arithmetic2/2
  Delay2/1 -> Multiport Switch1/1
  Delay1/1 -> AND/1, Block RAM/3(wr_en)
  Delay/1 -> Relational Operator/1, Block RAM/2(wr_addr)
  Constant1/1 -> Shift Arithmetic1/1
  Constant/1 -> Bit Concat/1
  Bitwise NOT/1 -> Bitwise AND/1
  Bit Slice/1 -> hps/1, Add/2
  AND/1 -> Delay2/1
  shift/1 -> Delay4/1
  mode/1 -> Multiport Switch/1
  address/1 -> Relational Operator/2, Delay/1, Block RAM/4(rd_addr)
  edge/1 -> Delay1/1
  Delay5/1 -> Multiport Switch1/3
  Shift Arithmetic/1 -> Bitwise OR/2
  Bit Concat/1 -> Shift Arithmetic/1
  Multiport Switch/1 -> Bit Concat/2
  Add/1 -> Multiport Switch/3
  Shift Arithmetic2/1 -> Bit Slice/1
  Bitwise AND/1 -> Bitwise OR/1
  Bitwise OR/1 -> Delay5/1, Block RAM/1(wr_data)
  Signal Specification/1 -> Multiport Switch1/2
  Multiport Switch1/1 -> Bitwise AND/2, Shift Arithmetic2/1
  Block RAM/1(rd_data) -> Signal Specification/1

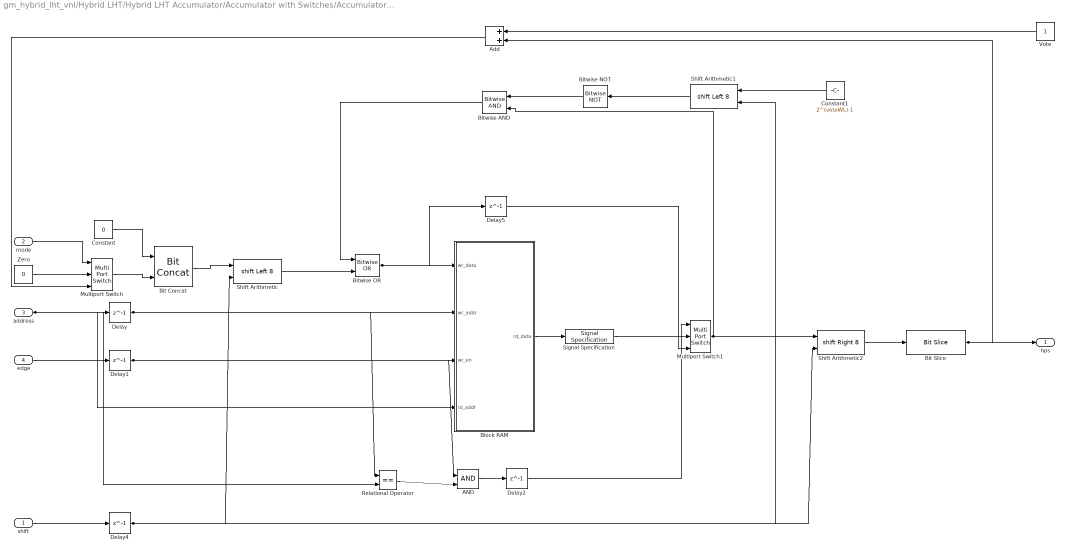
== system gm_hybrid_lht_vnl/Hybrid LHT/Hybrid LHT Accumulator/Accumulator with Switches/Accumulator_instance12 ==
  shift : Inport  OutDataTypeStr=fixdt(0, 6, 0)  PortDimensions=1  SampleTime=8.33333333333333e-09
  mode : Inport  Port=2  OutDataTypeStr=boolean  PortDimensions=1  SampleTime=8.33333333333333e-09
  address : Inport  Port=3  OutDataTypeStr=fixdt(0, 11, 0)  PortDimensions=1  SampleTime=8.33333333333333e-09
  edge : Inport  Port=4  OutDataTypeStr=boolean  PortDimensions=1  SampleTime=8.33333333333333e-09
  AND : Logic  IconShape=distinctive  AllPortsSameDT=off  OutDataTypeStr=boolean
  Add : Sum  OutDataTypeStr=fixdt(0, ceil(log2(maxRho*2)), 0)
  Bit Concat : hdlsllib/Logic and Bit Operations/Bit Concat  numInputs=2
      settings: SourceProductName=Simulink
  Bit Slice : hdlsllib/Logic and Bit Operations/Bit Slice  lidx=voteWL-1  ridx=0
  Bitwise AND : simulink/Logic and Bit Operations/Bitwise Operator  logicop=AND  UseBitMask=off  NumInputPorts=2  BitMask=bin2dec('11011001')  BitMaskRealWorld=Stored Integer
  Bitwise NOT : simulink/Logic and Bit Operations/Bitwise Operator  logicop=NOT  UseBitMask=off  BitMask=bin2dec('11011001')  BitMaskRealWorld=Stored Integer
  Bitwise OR : simulink/Logic and Bit Operations/Bitwise Operator  logicop=OR  UseBitMask=off  NumInputPorts=2  BitMask=bin2dec('11011001')  BitMaskRealWorld=Stored Integer
  Block RAM : Subsystem
  Constant : Constant  Value=0  OutDataTypeStr=fixdt(0, 36-voteWL, 0)  SampleTime=-1
  Constant1 : Constant  Value=2^(voteWL)-1  OutDataTypeStr=fixdt(0, 36, 0)  SampleTime=-1
  Delay{,1..2,4..5} (5 alike) : Delay  DelayLength=1
  Multiport Switch : MultiPortSwitch  DataPortOrder=Zero-based contiguous  Inputs=2  zeroidx=on
  Multiport Switch1 : MultiPortSwitch  DataPortOrder=Zero-based contiguous  Inputs=2  zeroidx=on
  Relational Operator : RelationalOperator  Operator===  OutDataTypeStr=boolean  RndMeth=Simplest
  Shift Arithmetic : ArithShift  BitShiftNumberSource=Input port  BitShiftNumber=8  BitShiftDirection=Left  DiagnosticForOORShift=Error
      settings: InputPortMap=u0,p1
  Shift Arithmetic1 : ArithShift  BitShiftNumberSource=Input port  BitShiftNumber=8  BitShiftDirection=Left  DiagnosticForOORShift=Error
      settings: InputPortMap=u0,p1
  Shift Arithmetic2 : ArithShift  BitShiftNumberSource=Input port  BitShiftNumber=8  BitShiftDirection=Right  DiagnosticForOORShift=Error
      settings: InputPortMap=u0,p1
  Signal Specification : SignalSpecification  OutDataTypeStr=fixdt(0, 36, 0)
  Vote : Constant  OutDataTypeStr=fixdt(0,1,0)  SampleTime=-1
  Zero : Constant  Value=0  OutDataTypeStr=fixdt(0,1,0)  SampleTime=-1
  hps : Outport
  wires:
  Zero/1 -> Multiport Switch/2
  Vote/1 -> Add/1
  Shift Arithmetic1/1 -> Bitwise NOT/1
  Relational Operator/1 -> AND/2
  Delay4/1 -> Shift Arithmetic1/2, Shift Arithmetic/2, Shift Arithmetic2/2
  Delay2/1 -> Multiport Switch1/1
  Delay1/1 -> AND/1, Block RAM/3(wr_en)
  Delay/1 -> Relational Operator/1, Block RAM/2(wr_addr)
  Constant1/1 -> Shift Arithmetic1/1
  Constant/1 -> Bit Concat/1
  Bitwise NOT/1 -> Bitwise AND/1
  Bit Slice/1 -> hps/1, Add/2
  AND/1 -> Delay2/1
  shift/1 -> Delay4/1
  mode/1 -> Multiport Switch/1
  address/1 -> Relational Operator/2, Delay/1, Block RAM/4(rd_addr)
  edge/1 -> Delay1/1
  Delay5/1 -> Multiport Switch1/3
  Shift Arithmetic/1 -> Bitwise OR/2
  Bit Concat/1 -> Shift Arithmetic/1
  Multiport Switch/1 -> Bit Concat/2
  Add/1 -> Multiport Switch/3
  Shift Arithmetic2/1 -> Bit Slice/1
  Bitwise AND/1 -> Bitwise OR/1
  Bitwise OR/1 -> Delay5/1, Block RAM/1(wr_data)
  Signal Specification/1 -> Multiport Switch1/2
  Multiport Switch1/1 -> Bitwise AND/2, Shift Arithmetic2/1
  Block RAM/1(rd_data) -> Signal Specification/1

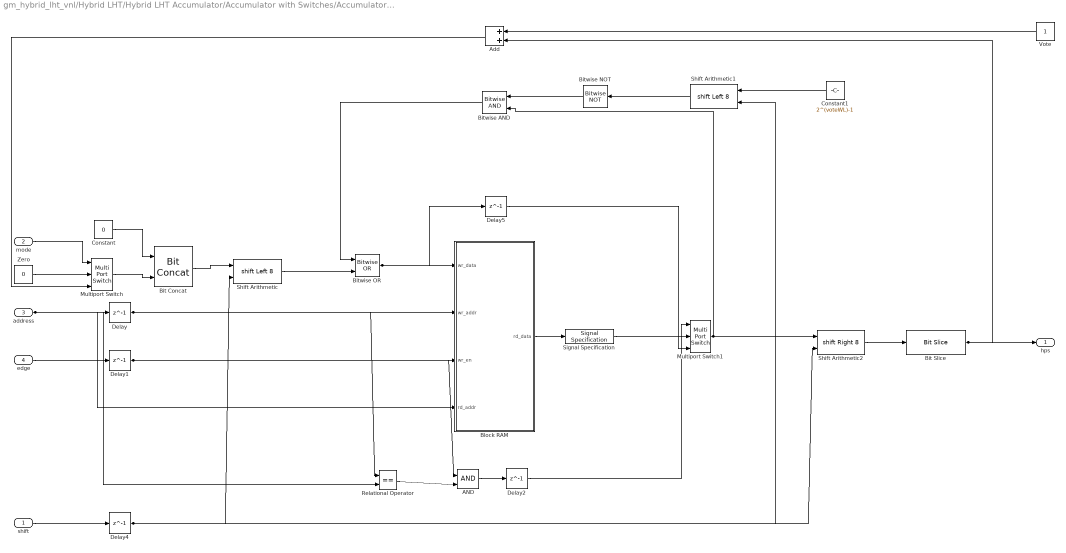
== system gm_hybrid_lht_vnl/Hybrid LHT/Hybrid LHT Accumulator/Accumulator with Switches/Accumulator_instance13 ==
  shift : Inport  OutDataTypeStr=fixdt(0, 6, 0)  PortDimensions=1  SampleTime=8.33333333333333e-09
  mode : Inport  Port=2  OutDataTypeStr=boolean  PortDimensions=1  SampleTime=8.33333333333333e-09
  address : Inport  Port=3  OutDataTypeStr=fixdt(0, 11, 0)  PortDimensions=1  SampleTime=8.33333333333333e-09
  edge : Inport  Port=4  OutDataTypeStr=boolean  PortDimensions=1  SampleTime=8.33333333333333e-09
  AND : Logic  IconShape=distinctive  AllPortsSameDT=off  OutDataTypeStr=boolean
  Add : Sum  OutDataTypeStr=fixdt(0, ceil(log2(maxRho*2)), 0)
  Bit Concat : hdlsllib/Logic and Bit Operations/Bit Concat  numInputs=2
      settings: SourceProductName=Simulink
  Bit Slice : hdlsllib/Logic and Bit Operations/Bit Slice  lidx=voteWL-1  ridx=0
  Bitwise AND : simulink/Logic and Bit Operations/Bitwise Operator  logicop=AND  UseBitMask=off  NumInputPorts=2  BitMask=bin2dec('11011001')  BitMaskRealWorld=Stored Integer
  Bitwise NOT : simulink/Logic and Bit Operations/Bitwise Operator  logicop=NOT  UseBitMask=off  BitMask=bin2dec('11011001')  BitMaskRealWorld=Stored Integer
  Bitwise OR : simulink/Logic and Bit Operations/Bitwise Operator  logicop=OR  UseBitMask=off  NumInputPorts=2  BitMask=bin2dec('11011001')  BitMaskRealWorld=Stored Integer
  Block RAM : Subsystem
  Constant : Constant  Value=0  OutDataTypeStr=fixdt(0, 36-voteWL, 0)  SampleTime=-1
  Constant1 : Constant  Value=2^(voteWL)-1  OutDataTypeStr=fixdt(0, 36, 0)  SampleTime=-1
  Delay{,1..2,4..5} (5 alike) : Delay  DelayLength=1
  Multiport Switch : MultiPortSwitch  DataPortOrder=Zero-based contiguous  Inputs=2  zeroidx=on
  Multiport Switch1 : MultiPortSwitch  DataPortOrder=Zero-based contiguous  Inputs=2  zeroidx=on
  Relational Operator : RelationalOperator  Operator===  OutDataTypeStr=boolean  RndMeth=Simplest
  Shift Arithmetic : ArithShift  BitShiftNumberSource=Input port  BitShiftNumber=8  BitShiftDirection=Left  DiagnosticForOORShift=Error
      settings: InputPortMap=u0,p1
  Shift Arithmetic1 : ArithShift  BitShiftNumberSource=Input port  BitShiftNumber=8  BitShiftDirection=Left  DiagnosticForOORShift=Error
      settings: InputPortMap=u0,p1
  Shift Arithmetic2 : ArithShift  BitShiftNumberSource=Input port  BitShiftNumber=8  BitShiftDirection=Right  DiagnosticForOORShift=Error
      settings: InputPortMap=u0,p1
  Signal Specification : SignalSpecification  OutDataTypeStr=fixdt(0, 36, 0)
  Vote : Constant  OutDataTypeStr=fixdt(0,1,0)  SampleTime=-1
  Zero : Constant  Value=0  OutDataTypeStr=fixdt(0,1,0)  SampleTime=-1
  hps : Outport
  wires:
  Zero/1 -> Multiport Switch/2
  Vote/1 -> Add/1
  Shift Arithmetic1/1 -> Bitwise NOT/1
  Relational Operator/1 -> AND/2
  Delay4/1 -> Shift Arithmetic1/2, Shift Arithmetic/2, Shift Arithmetic2/2
  Delay2/1 -> Multiport Switch1/1
  Delay1/1 -> AND/1, Block RAM/3(wr_en)
  Delay/1 -> Relational Operator/1, Block RAM/2(wr_addr)
  Constant1/1 -> Shift Arithmetic1/1
  Constant/1 -> Bit Concat/1
  Bitwise NOT/1 -> Bitwise AND/1
  Bit Slice/1 -> hps/1, Add/2
  AND/1 -> Delay2/1
  shift/1 -> Delay4/1
  mode/1 -> Multiport Switch/1
  address/1 -> Relational Operator/2, Delay/1, Block RAM/4(rd_addr)
  edge/1 -> Delay1/1
  Delay5/1 -> Multiport Switch1/3
  Shift Arithmetic/1 -> Bitwise OR/2
  Bit Concat/1 -> Shift Arithmetic/1
  Multiport Switch/1 -> Bit Concat/2
  Add/1 -> Multiport Switch/3
  Shift Arithmetic2/1 -> Bit Slice/1
  Bitwise AND/1 -> Bitwise OR/1
  Bitwise OR/1 -> Delay5/1, Block RAM/1(wr_data)
  Signal Specification/1 -> Multiport Switch1/2
  Multiport Switch1/1 -> Bitwise AND/2, Shift Arithmetic2/1
  Block RAM/1(rd_data) -> Signal Specification/1
